simulink model "fuzzy_simulink_sim_1"  (R2015b)
settings: Solver=VariableStepAuto  StartTime=0.0  StopTime=200  RelTol=1e-3
libraries: fuzblock x1
settings Model: Creator=giorgos  LastModifiedBy=giorgos

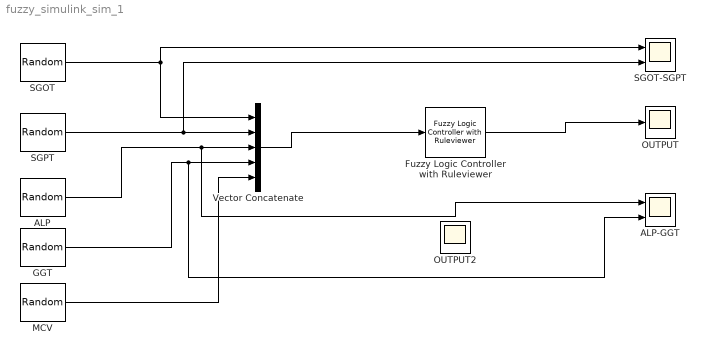
== system fuzzy_simulink_sim_1 ==
  "ALP " : UniformRandomNumber  Minimum=30  Maximum=200  Seed=3  SampleTime=5
  ALP-GGT : Scope  NumInputPorts=2
  Fuzzy Logic Controller with Ruleviewer : fuzblock/Fuzzy Logic  Controller  with Ruleviewer  fismatrix=a  Ts=5
  "GGT " : UniformRandomNumber  Minimum=10  Maximum=80  Seed=4  SampleTime=5
  MCV : UniformRandomNumber  Minimum=80  Maximum=100  Seed=5  SampleTime=5
  OUTPUT : Scope
  OUTPUT2 : Scope
  "SGOT " : UniformRandomNumber  Minimum=10  Maximum=75  SampleTime=5
  SGOT-SGPT : Scope  NumInputPorts=2
  SGPT : UniformRandomNumber  Minimum=5  Maximum=70  Seed=1  SampleTime=5
  Vector Concatenate : Concatenate  NumInputs=5
  wires:
  MCV/1 -> Vector Concatenate/5
  "GGT "/1 -> ALP-GGT/2, Vector Concatenate/4
  "ALP "/1 -> ALP-GGT/1, Vector Concatenate/3
  Vector Concatenate/1 -> Fuzzy Logic Controller with Ruleviewer/1
  Fuzzy Logic Controller with Ruleviewer/1 -> OUTPUT/1
  SGPT/1 -> SGOT-SGPT/2, Vector Concatenate/2
  "SGOT "/1 -> SGOT-SGPT/1, Vector Concatenate/1
